simulink model "velocity_tracking_low_damping"  (R2018b)
settings: Solver=ode8  StartTime=0.0  StopTime=14  FixedStep=0.05  RelTol=1e-3
settings Model: Creator=suvo.ganguli  LastModifiedBy=suvo.ganguli

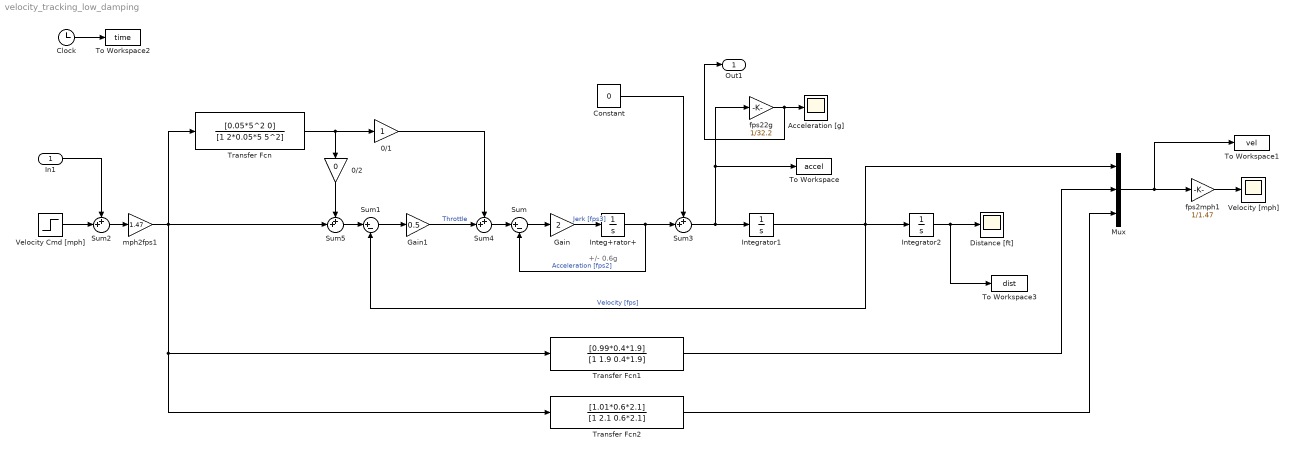
== system velocity_tracking_low_damping ==
  note: +/- 0.6g
  In1 : Inport
  0/1 : Gain
  0/2 : Gain  Gain=0
  Acceleration [g] : Scope
  Clock : Clock
  Constant : Constant  Value=0
  Distance [ft] : Scope
  Gain : Gain  Gain=2
  Gain1 : Gain  Gain=0.5
  Integ+rator+ : Integrator  LimitOutput=on  UpperSaturationLimit=0.6*32.2  LowerSaturationLimit=-0.6*32.2
  Integrator1 : Integrator
  Integrator2 : Integrator
  Mux : Mux  Inputs=3
  Sum : Sum  Inputs=|+-
  Sum1 : Sum  Inputs=|+-
  Sum{2..5} (4 alike) : Sum  Inputs=++|
  To Workspace : ToWorkspace  VariableName=accel  SampleTime=-1
  To Workspace1 : ToWorkspace  VariableName=vel  SampleTime=-1
  To Workspace2 : ToWorkspace  VariableName=time  SampleTime=-1
  To Workspace3 : ToWorkspace  VariableName=dist  SampleTime=-1
  Transfer Fcn : TransferFcn  Numerator=[0.05*5^2 0]  Denominator=[1 2*0.05*5 5^2]
  Transfer Fcn1 : TransferFcn  Numerator=[0.99*0.4*1.9]  Denominator=[1 1.9 0.4*1.9]
  Transfer Fcn2 : TransferFcn  Numerator=[1.01*0.6*2.1]  Denominator=[1 2.1 0.6*2.1]
  Velocity [mph] : Scope
  Velocity Cmd [mph] : Step  Time=0  After=45  SampleTime=0
  fps22g : Gain  Gain=1/32.2
  fps2mph1 : Gain  Gain=1/1.47
  mph2fps1 : Gain  Gain=1.47
  Out1 : Outport
  wires:
  Sum/1 -> Gain/1
  Gain/1 -> Integ+rator+/1  "Jerk [fps3]"
  Sum1/1 -> Gain1/1
  Integrator1/1 -> Sum1/2, Integrator2/1, Mux/1  "Velocity [fps]"
  Integrator2/1 -> To Workspace3/1, Distance [ft]/1
  fps22g/1 -> Out1/1, Acceleration [g]/1
  Clock/1 -> To Workspace2/1
  Integ+rator+/1 -> Sum/2, Sum3/2  "Acceleration [fps2]"
  Mux/1 -> To Workspace1/1, fps2mph1/1
  Transfer Fcn1/1 -> Mux/2
  fps2mph1/1 -> Velocity [mph]/1
  Transfer Fcn2/1 -> Mux/3
  Sum3/1 -> To Workspace/1, fps22g/1, Integrator1/1
  Velocity Cmd [mph]/1 -> Sum2/2
  Sum2/1 -> mph2fps1/1
  In1/1 -> Sum2/1
  mph2fps1/1 -> Sum5/2, Transfer Fcn1/1, Transfer Fcn2/1, Transfer Fcn/1
  Constant/1 -> Sum3/1
  Transfer Fcn/1 -> 0/2/1, 0/1/1
  Sum4/1 -> Sum/1
  Gain1/1 -> Sum4/2  "Throttle"
  Sum5/1 -> Sum1/1
  0/1/1 -> Sum4/1
  0/2/1 -> Sum5/1
